simulink model "Ui_1V_step_response"  (R2013a)
settings: Solver=ode45  StartTime=0.0  StopTime=15  FixedStep=0.005  RelTol=1e-3
undefined symbols (not defined in the file or in its folder): B, Jeff1, Jeff2, Km, qInitial, R, r
settings Model: Creator=Mylene  LastModifiedBy=user
settings DataIOCC: SignalLoggingSaveFormat=ModelDataLogs
settings OptimizationCC: ExpressionDepthLimit=2147483647
settings DebuggingCC: FcnCallInpInsideContextMsg=UseLocalSettings
settings GRTTargetCC: CombineOutputUpdateFcns=off  GRTInterface=on

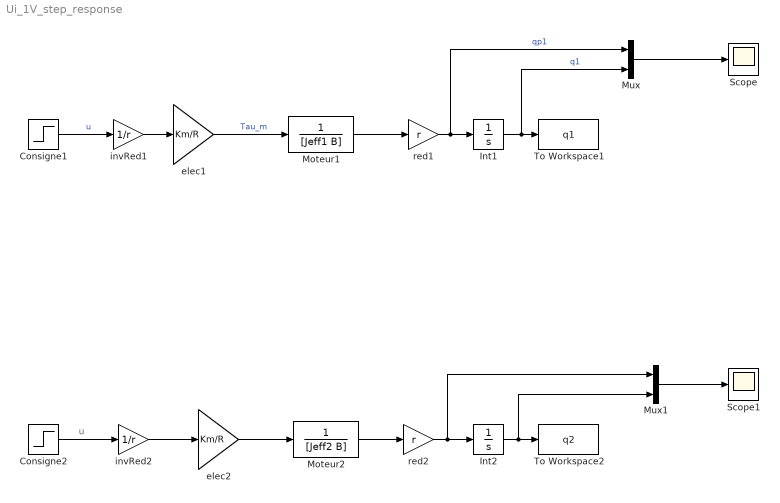
== system Ui_1V_step_response ==
  note: u
  Consigne1 : Step  SampleTime=0
  Consigne2 : Step  SampleTime=0
  Int1 : Integrator  InitialCondition=qInitial
  Int2 : Integrator  InitialCondition=qInitial
  Moteur1 : TransferFcn  Denominator=[Jeff1 B]
  Moteur2 : TransferFcn  Denominator=[Jeff2 B]
  Mux : Mux  Inputs=2
  Mux1 : Mux  Inputs=2
  Scope : Scope
  Scope1 : Scope
  To Workspace1 : ToWorkspace  VariableName=q1  SampleTime=-1
  To Workspace2 : ToWorkspace  VariableName=q2  SampleTime=-1
  elec1 : Gain  Gain=Km/R
  elec2 : Gain  Gain=Km/R
  invRed1 : Gain  Gain=1/r
  invRed2 : Gain  Gain=1/r
  red1 : Gain  Gain=r
  red2 : Gain  Gain=r
  wires:
  elec1/1 -> Moteur1/1  "Tau_m"
  elec2/1 -> Moteur2/1
  Consigne2/1 -> invRed2/1
  red1/1 -> Mux/1, Int1/1  "qp1"
  Moteur1/1 -> red1/1
  Int1/1 -> Mux/2, To Workspace1/1  "q1"
  Moteur2/1 -> red2/1
  red2/1 -> Mux1/1, Int2/1
  Int2/1 -> Mux1/2, To Workspace2/1
  invRed1/1 -> elec1/1
  Consigne1/1 -> invRed1/1  "u"
  invRed2/1 -> elec2/1
  Mux/1 -> Scope/1
  Mux1/1 -> Scope1/1
